simulink model "combinedConverter"  (R2025b)
settings: Solver=VariableStepAuto  StartTime=0.0  StopTime=10.0  RelTol=1e-3

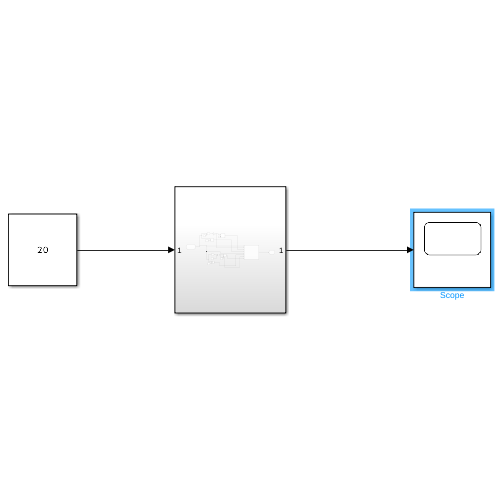
[thumbnail: Simulink's stored preview of the top-level diagram]
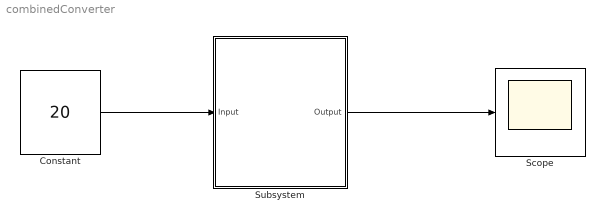
== system combinedConverter ==
  Constant : Constant  Value=20
  Scope : Scope
      settings: ActiveDisplayYMinimum=-73.45875  ActiveDisplayYMaximum=594.46208333333345
  Subsystem : Subsystem
  wires:
  Subsystem/1(Output) -> Scope/1
  Constant/1 -> Subsystem/1(Input)

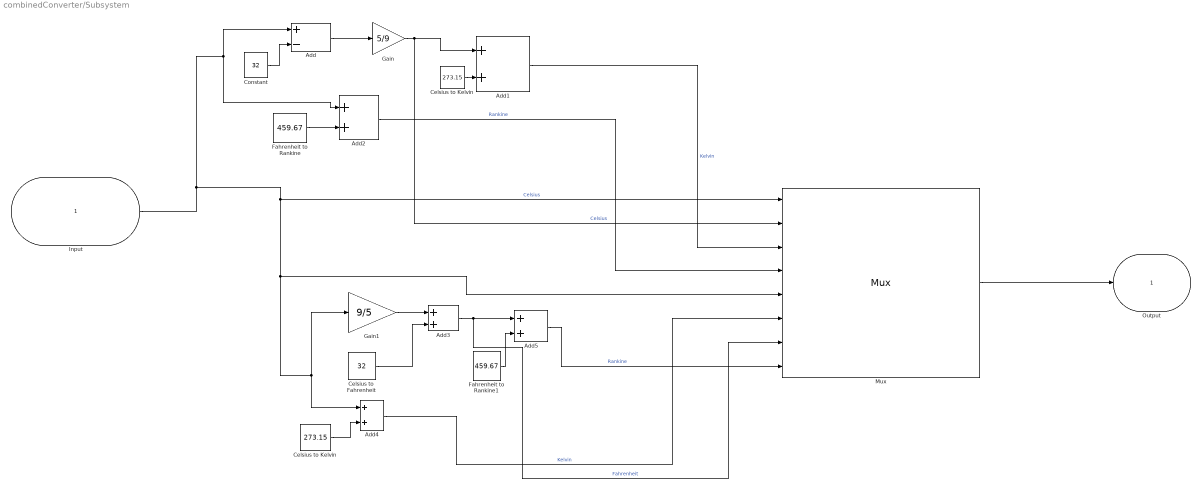
== system combinedConverter/Subsystem ==
  Input : Inport
  Add : Sum  Inputs=+-
  Add{1..5} (5 alike) : Sum
  Celsius to Fahrenheit : Constant  Value=32
  Celsius to Kelvin : Constant  Value=273.15
  "Celsius to Kelvin " : Constant  Value=273.15
  Constant : Constant  Value=32
  Fahrenheit to Rankine : Constant  Value=459.67
  Fahrenheit to Rankine1 : Constant  Value=459.67
  Gain : Gain  Gain=5/9
  Gain1 : Gain  Gain=9/5
  Mux : Mux  Inputs=8
  Output : Outport
  wires:
  Add1/1 -> Mux/3  "Kelvin"
  Constant/1 -> Add/2
  Fahrenheit to Rankine/1 -> Add2/2
  Add/1 -> Gain/1
  Gain/1 -> Mux/2, Add1/1  "Celsius"
  Celsius to Kelvin/1 -> Add1/2
  Add2/1 -> Mux/4  "Rankine"
  Add4/1 -> Mux/6  "Kelvin"
  Add5/1 -> Mux/8  "Rankine"
  Celsius to Fahrenheit/1 -> Add3/2
  Gain1/1 -> Add3/1
  "Celsius to Kelvin "/1 -> Add4/2
  Input/1 -> Mux/1, Gain1/1, Add4/1, Mux/5, Add2/1, Add/1  "Celsius"
  Add3/1 -> Mux/7, Add5/1  "Fahrenheit"
  Fahrenheit to Rankine1/1 -> Add5/2
  Mux/1 -> Output/1
